simulink model "battery_simulation_varsion1"  (R2026a)
settings: Solver=ode23t  StopTime=1450  MaxStep=10  RelTol=1e-4
settings Model: Creator=shlom  LastModifiedBy=shlom
settings DebuggingCC: AlgebraicLoopMsg=error
settings SimscapeCC: SimscapeLogType=none

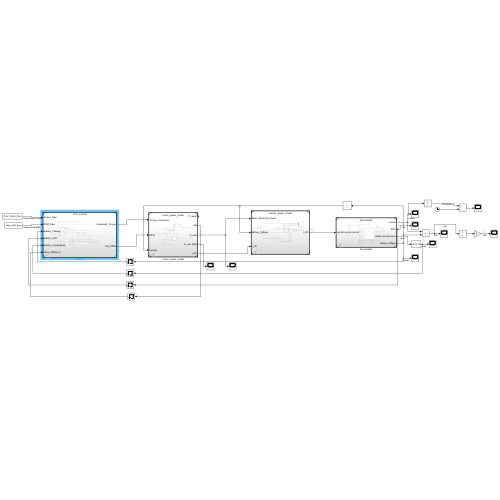
[thumbnail: Simulink's stored preview of the top-level diagram]
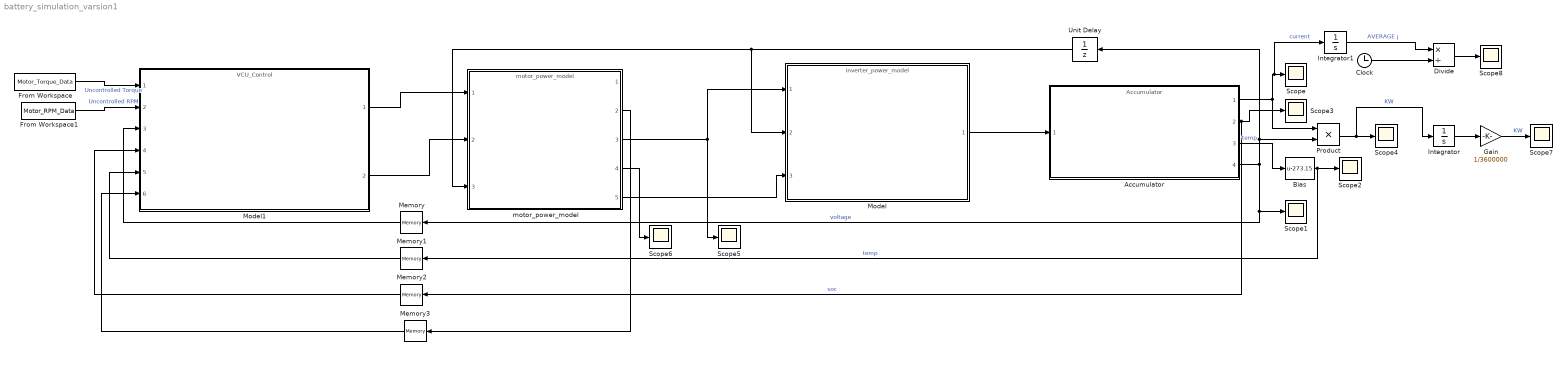
== system battery_simulation_varsion1 ==
  Accumulator : ModelReference  ModelNameDialog=Accumulator.slx  SimulationMode=Normal  ModelReferenceVersion=1.17
  Bias : Bias  Bias=-273.15  SaturateOnIntegerOverflow=off
  Clock : Clock
  Divide : Product  Inputs=*/
  From Workspace : FromWorkspace  VariableName=Motor_Torque_Data
  From Workspace1 : FromWorkspace  VariableName=Motor_RPM_Data
  Gain : Gain  Gain=1/3600000
  Integrator : Integrator
  Integrator1 : Integrator
  Memory{,1..3} (4 alike) : Memory
  Model : ModelReference  ModelNameDialog=inverter_power_model.slx  SimulationMode=Normal  ModelReferenceVersion=1.3
  Model1 : ModelReference  ModelNameDialog=VCU_Control.slx  SimulationMode=Normal  ModelReferenceVersion=1.13
  Product : Product
  Scope{,1..8} (9 alike) : Scope
      Scope settings: ActiveDisplayYMinimum=-47.367906085464426  ActiveDisplayYMaximum=197.46555766725808
      Scope1 settings: ActiveDisplayYMinimum=360.18184805466427  ActiveDisplayYMaximum=622.6213615219998
      Scope2 settings: ActiveDisplayYMinimum=-81.189790252368965  ActiveDisplayYMaximum=180.70088174511679  DataLoggingVariableName=ScopeData2
      Scope3 settings: ActiveDisplayYMinimum=0.17478672739498458  ActiveDisplayYMaximum=0.24087547869632286  DataLoggingVariableName=ScopeData3
      Scope4 settings: ActiveDisplayYMinimum=-27726.740617022231  ActiveDisplayYMaximum=85970.516714487312  DataLoggingVariableName=ScopeData4
      Scope5 settings: ActiveDisplayYMinimum=-50239.389503984  ActiveDisplayYMaximum=141692.16220263948  DataLoggingVariableName=ScopeData5
      Scope6 settings: ActiveDisplayYMinimum=-212.69341659569056  ActiveDisplayYMaximum=732.604235795713  DataLoggingVariableName=ScopeData6
      Scope7 settings: ActiveDisplayYMinimum=7.6953488796673906  ActiveDisplayYMaximum=8.3163968450110541  DataLoggingVariableName=ScopeData7
      Scope8 settings: ActiveDisplayYMinimum=-7.78539846634628  ActiveDisplayYMaximum=60.000804956238213  DataLoggingVariableName=ScopeData8
  Unit Delay : UnitDelay  InitialCondition=588  SampleTime=-1
  motor_power_model : ModelReference  ModelNameDialog=motor_power_model.slx  SimulationMode=Normal  ModelReferenceVersion=1.3
  wires:
  Model1/1 -> motor_power_model/1
  Model1/2 -> motor_power_model/2
  motor_power_model/4 -> Scope6/1
  Unit Delay/1 -> Model/2, motor_power_model/3
  Model/1 -> Accumulator/1
  Accumulator/1 -> Integrator1/1, Scope/1, Product/1  "current"
  From Workspace/1 -> Model1/1  "Uncontrolled Torque"
  From Workspace1/1 -> Model1/2  "Uncontrolled RPM"
  Accumulator/2 -> Memory2/1, Scope3/1  "soc"
  Accumulator/3 -> Bias/1  "temp"
  Product/1 -> Integrator/1, Scope4/1  "KW"
  Accumulator/4 -> Memory/1, Scope1/1, Product/2, Unit Delay/1  "voltage"
  motor_power_model/3 -> Model/1, Scope5/1
  Integrator/1 -> Gain/1
  Gain/1 -> Scope7/1  "KW"
  Bias/1 -> Memory1/1, Scope2/1  "temp"
  motor_power_model/5 -> Model/3
  Memory/1 -> Model1/3
  Memory1/1 -> Model1/5
  Memory2/1 -> Model1/4
  motor_power_model/2 -> Memory3/1
  Memory3/1 -> Model1/6
  Integrator1/1 -> Divide/1  "AVERAGE ן"
  Clock/1 -> Divide/2
  Divide/1 -> Scope8/1
